simulink model "x25_CPM_130_Causal_Vitesse"  (R2024b)
settings: Solver=VariableStepAuto  StartTime=0.0  StopTime=.8  RelTol=1e-3
InitFcn:
  | run("parametres.m")
  | %data = lire_csv_rc4("Echelon_CH_P50_HG.csv")
values from neighbouring files (symbols this model uses):
  Cfs = 0.003    [parametres.m]
  fv = 2.e-6    (= 2e-06)    [parametres.m]
  ISAT = 1.2    [parametres.m]
  Jm = Jm+Jr    (= 1.6219e-06)    [parametres.m]
  Kcm = 25.6e-3    (= 0.0256)    [parametres.m]
  KCou_I = 1000    [parametres.m]
  KCou_P = 1000    [parametres.m]
  Kem = 1/(373 *2*pi/60)    (= 0.0256013313285)    [parametres.m]
  KVit_I = 90    [parametres.m]
  KVit_P = 470    [parametres.m]
  Lm = 0.278e-3    (= 0.000278)    [parametres.m]
  Rm = 2.14    [parametres.m]
  Unom = 24    [parametres.m]
settings Model: Creator=xavier.pessoles2  LastModifiedBy=xpess

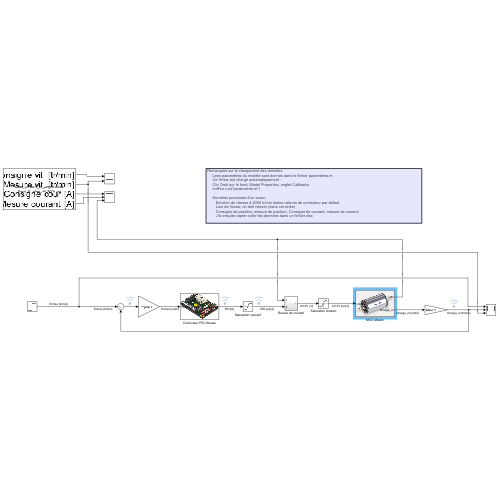
[thumbnail: Simulink's stored preview of the top-level diagram]
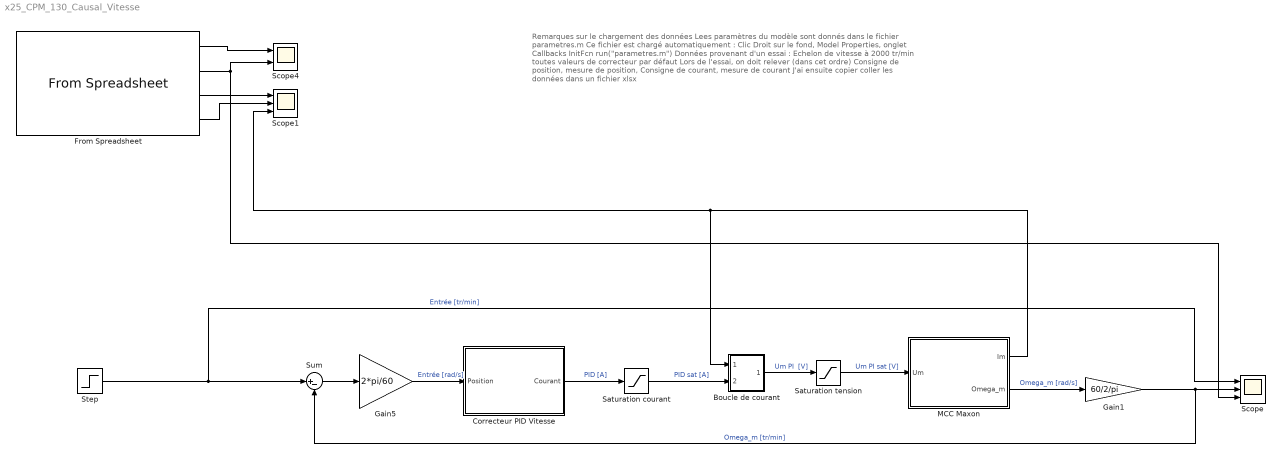
== system x25_CPM_130_Causal_Vitesse ==
  note: Remarques sur le chargement des données
      |      Lees paramètres du modèle sont donnés dans le fichier parametres.m
      |      Ce fichier est chargé automatiquement :
      |      Clic Droit sur le fond, Model Properties, onglet Callbacks
      |      InitFcn run("parametres.m")
      |
      |      Données provenant d'un essai :
      |         Echelon de vitesse à 2000 tr/min toutes valeurs de correcteur par défaut
      |         Lors de l'essai, on doit relever (dans cet ordre)
      |         Consigne de position, mesure de position, Consigne de courant, mesure de courant
      |         J'ai ensuite copier coller les données dans un fichier xlsx
  Boucle de courant : Subsystem
  Correcteur PID Vitesse : Subsystem
      mask Display: image('EPOS.png');
  From Spreadsheet : FromSpreadsheet  FileName=Essai_Echelon_Vit_2000mm.xlsx  SheetName=Essai_Echelon_Vit_2000mm
  Gain1 : Gain  Gain=60/2/pi
  Gain5 : Gain  Gain=2*pi/60
  MCC Maxon : Subsystem
      mask Display: image('MCC.png');
  Saturation courant : Saturate  UpperLimit=ISAT  LowerLimit=-ISAT
  Saturation tension : Saturate  UpperLimit=Unom  LowerLimit=-Unom
  Scope : Scope  NumInputPorts=3
  Scope1 : Scope  NumInputPorts=3
  Scope4 : Scope  NumInputPorts=2
  Step : Step  Time=.08  After=2000  SampleTime=0
  Sum : Sum  Inputs=|+-
  wires:
  Sum/1 -> Gain5/1
  MCC Maxon/1(Im) -> Boucle de courant/1(In1), Scope1/3
  Correcteur PID Vitesse/1(Courant) -> Saturation courant/1  "PID [A]"
  Boucle de courant/1(Out1) -> Saturation tension/1  "Um PI  [V]"
  Saturation tension/1 -> MCC Maxon/1(Um)  "Um PI sat [V]"
  Saturation courant/1 -> Boucle de courant/2(In2)  "PID sat [A]"
  Step/1 -> Sum/1, Scope/1  "Entrée [tr/min]"
  Gain5/1 -> Correcteur PID Vitesse/1(Position)  "Entrée [rad/s]"
  From Spreadsheet/1 -> Scope4/1
  MCC Maxon/2(Omega_m) -> Gain1/1  "Omega_m [rad/s]"
  Gain1/1 -> Scope/2, Sum/2  "Omega_m [tr/min]"
  From Spreadsheet/2 -> Scope4/2, Scope/3
  From Spreadsheet/3 -> Scope1/1
  From Spreadsheet/4 -> Scope1/2

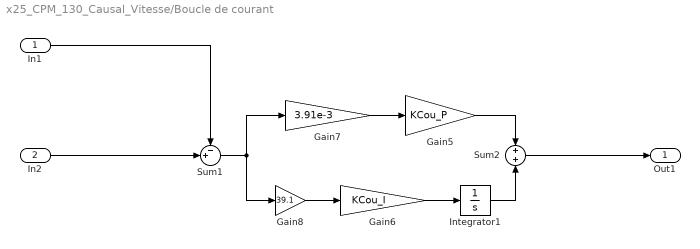
== system x25_CPM_130_Causal_Vitesse/Boucle de courant ==
  In1 : Inport
  In2 : Inport  Port=2
  Gain5 : Gain  Gain=KCou_P
  Gain6 : Gain  Gain=KCou_I
  Gain7 : Gain  Gain=3.91e-3
  Gain8 : Gain  Gain=39.1
  Integrator1 : Integrator
  Sum1 : Sum  Inputs=-+|
  Sum2 : Sum  Inputs=+|+
  Out1 : Outport
  wires:
  Sum1/1 -> Gain7/1, Gain8/1
  Gain5/1 -> Sum2/1
  Sum2/1 -> Out1/1
  Integrator1/1 -> Sum2/2
  Gain8/1 -> Gain6/1
  In1/1 -> Sum1/1
  Gain7/1 -> Gain5/1
  Gain6/1 -> Integrator1/1
  In2/1 -> Sum1/2

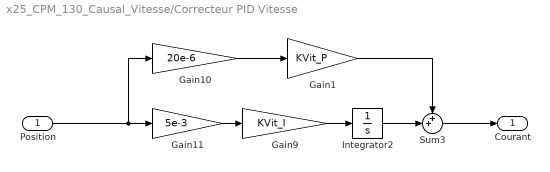
== system x25_CPM_130_Causal_Vitesse/Correcteur PID Vitesse ==
  Position : Inport
  Gain1 : Gain  Gain=KVit_P
  Gain10 : Gain  Gain=20e-6
  Gain11 : Gain  Gain=5e-3
  Gain9 : Gain  Gain=KVit_I
  Integrator2 : Integrator
  Sum3 : Sum  Inputs=++|
  Courant : Outport
  wires:
  Gain1/1 -> Sum3/1
  Position/1 -> Gain10/1, Gain11/1
  Gain9/1 -> Integrator2/1
  Sum3/1 -> Courant/1
  Integrator2/1 -> Sum3/2
  Gain10/1 -> Gain1/1
  Gain11/1 -> Gain9/1

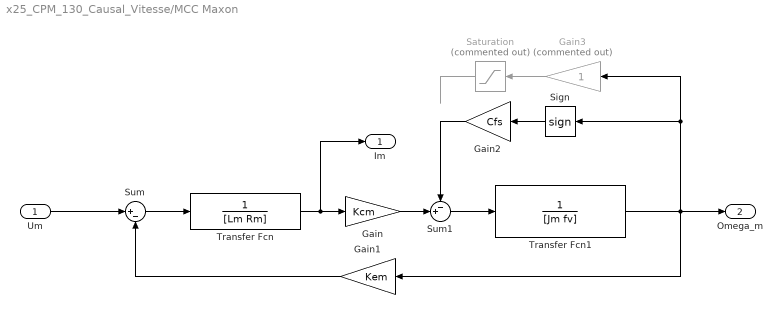
== system x25_CPM_130_Causal_Vitesse/MCC Maxon ==
  Um : Inport
  Gain : Gain  Gain=Kcm
  Gain1 : Gain  Gain=Kem
  Gain2 : Gain  Gain=Cfs
  Gain3 : Gain  Commented=on
  Saturation : Saturate  Commented=on  UpperLimit=Cfs  LowerLimit=-Cfs
  Sign : Signum
  Sum : Sum  Inputs=|+-
  Sum1 : Sum  Inputs=-+|
  Transfer Fcn : TransferFcn  Denominator=[Lm Rm]
  Transfer Fcn1 : TransferFcn  Denominator=[Jm fv]
  Im : Outport
  Omega_m : Outport  Port=2
  wires:
  Transfer Fcn/1 -> Im/1, Gain/1
  Transfer Fcn1/1 -> Sign/1, Gain3/1, Omega_m/1, Gain1/1
  Gain1/1 -> Sum/2
  Um/1 -> Sum/1
  Sum/1 -> Transfer Fcn/1
  Gain/1 -> Sum1/2
  Sum1/1 -> Transfer Fcn1/1
  Sign/1 -> Gain2/1
  Gain3/1 -> Saturation/1
  Saturation/1 -> ?
  Gain2/1 -> Sum1/1
